simulink model "OutputMVA"  (Simulink 8.7)
settings: Solver=ode45  StartTime=0.0  StopTime=10.0  RelTol=1e-3
undefined symbols (not defined in the file or in its folder): sMP
(part 3 of 3)

== system OutputMVA/OutputMVA_ACM/AMA_Filter ==
  NOx_gas_in : Inport
  Gain : Gain
  NOx_filtered : Outport
  wires:
  Gain/1 -> NOx_filtered/1
  NOx_gas_in/1 -> Gain/1

== system OutputMVA/OutputMVA_ACM/AMA_Filter1 ==
  NOx_gas_in : Inport
  Gain : Gain
  NOx_filtered : Outport
  wires:
  Gain/1 -> NOx_filtered/1
  NOx_gas_in/1 -> Gain/1

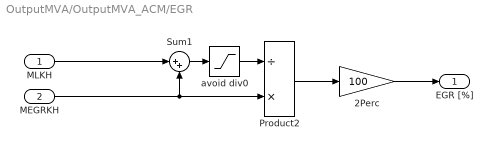
== system OutputMVA/OutputMVA_ACM/EGR ==
  MLKH : Inport
  MEGRKH : Inport  Port=2
  2Perc : Gain  Gain=100
  Product2 : Product  Inputs=/*  RndMeth=Zero
  Sum1 : Sum  Inputs=|++
  avoid div0 : Saturate  UpperLimit=inf  LowerLimit=0.000001
  "EGR [%] " : Outport
  wires:
  avoid div0/1 -> Product2/1
  2Perc/1 -> "EGR [%] "/1
  Sum1/1 -> avoid div0/1
  MLKH/1 -> Sum1/1
  MEGRKH/1 -> Product2/2, Sum1/2
  Product2/1 -> 2Perc/1

== system OutputMVA/OutputMVA_ACM/abs2rel_1 ==
  pressure_absolute : Inport
  Sum : Sum  Inputs=|+-
  pressure_relative : Outport
  wires:
  pressure_absolute/1 -> Sum/1
  Sum/1 -> pressure_relative/1
  [acm_OutputMVA_PressureReference] -> Sum/2

== system OutputMVA/OutputMVA_ACM/abs2rel_11 ==
  pressure_absolute : Inport
  Sum : Sum  Inputs=|+-
  pressure_relative : Outport
  wires:
  [acm_OutputMVA_PressureReference] -> Sum/2
  Sum/1 -> pressure_relative/1
  pressure_absolute/1 -> Sum/1

== system OutputMVA/OutputMVA_ACM/abs2rel_13 ==
  pressure_absolute : Inport
  Sum : Sum  Inputs=|+-
  pressure_relative : Outport
  wires:
  pressure_absolute/1 -> Sum/1
  Sum/1 -> pressure_relative/1
  [acm_OutputMVA_PressureReference] -> Sum/2

== system OutputMVA/OutputMVA_ACM/abs2rel_2 ==
  pressure_absolute : Inport
  Sum : Sum  Inputs=|+-
  pressure_relative : Outport
  wires:
  [acm_OutputMVA_PressureReference] -> Sum/2
  Sum/1 -> pressure_relative/1
  pressure_absolute/1 -> Sum/1

== system OutputMVA/OutputMVA_ACM/abs2rel_3 ==
  pressure_absolute : Inport
  Sum : Sum  Inputs=|+-
  pressure_relative : Outport
  wires:
  [acm_OutputMVA_PressureReference] -> Sum/2
  Sum/1 -> pressure_relative/1
  pressure_absolute/1 -> Sum/1

== system OutputMVA/OutputMVA_ACM/abs2rel_4 ==
  pressure_absolute : Inport
  Sum : Sum  Inputs=|+-
  pressure_relative : Outport
  wires:
  pressure_absolute/1 -> Sum/1
  Sum/1 -> pressure_relative/1
  [acm_OutputMVA_PressureReference] -> Sum/2

== system OutputMVA/OutputMVA_ACM/abs2rel_5 ==
  pressure_absolute : Inport
  Sum : Sum  Inputs=|+-
  pressure_relative : Outport
  wires:
  pressure_absolute/1 -> Sum/1
  Sum/1 -> pressure_relative/1
  [acm_OutputMVA_PressureReference] -> Sum/2

== system OutputMVA/OutputMVA_ACM/abs2rel_6 ==
  pressure_absolute : Inport
  Sum : Sum  Inputs=|+-
  pressure_relative : Outport
  wires:
  [acm_OutputMVA_PressureReference] -> Sum/2
  Sum/1 -> pressure_relative/1
  pressure_absolute/1 -> Sum/1

== system OutputMVA/OutputMVA_ACM/abs2rel_7 ==
  pressure_absolute : Inport
  Sum : Sum  Inputs=|+-
  pressure_relative : Outport
  wires:
  [acm_OutputMVA_PressureReference] -> Sum/2
  Sum/1 -> pressure_relative/1
  pressure_absolute/1 -> Sum/1

== system OutputMVA/OutputMVA_ACM/abs2rel_8 ==
  pressure_absolute : Inport
  Sum : Sum  Inputs=|+-
  pressure_relative : Outport
  wires:
  pressure_absolute/1 -> Sum/1
  Sum/1 -> pressure_relative/1
  [acm_OutputMVA_PressureReference] -> Sum/2

== system OutputMVA/OutputMVA_ACM/abs2rel_9 ==
  pressure_absolute : Inport
  Sum : Sum  Inputs=|+-
  pressure_relative : Outport
  wires:
  pressure_absolute/1 -> Sum/1
  Sum/1 -> pressure_relative/1
  [acm_OutputMVA_PressureReference] -> Sum/2

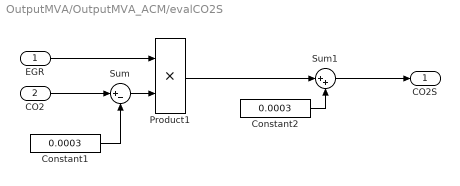
== system OutputMVA/OutputMVA_ACM/evalCO2S ==
  EGR : Inport
  CO2 : Inport  Port=2
  Constant1 : Constant  Value=0.0003
  Constant2 : Constant  Value=0.0003
  Product1 : Product  RndMeth=Zero
  Sum : Sum  Inputs=|+-
  Sum1 : Sum  Inputs=|++
  CO2S : Outport
  wires:
  EGR/1 -> Product1/1
  CO2/1 -> Sum/1
  Sum/1 -> Product1/2
  Constant1/1 -> Sum/2
  Product1/1 -> Sum1/1
  Constant2/1 -> Sum1/2
  Sum1/1 -> CO2S/1

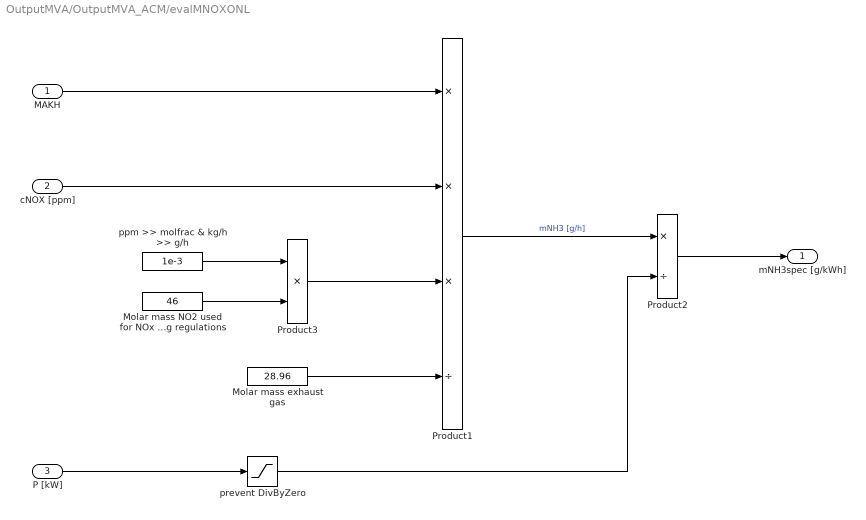
== system OutputMVA/OutputMVA_ACM/evalMNOXONL ==
  MAKH : Inport
  cNOX [ppm] : Inport  Port=2
  P [kW] : Inport  Port=3
  Molar mass NO2 used for NOx according regulations : Constant  Value=46
  Molar mass exhaust gas : Constant  Value=28.96
  Product1 : Product  Inputs=***/  RndMeth=Zero
  Product2 : Product  Inputs=*/  RndMeth=Zero
  Product3 : Product  RndMeth=Zero
  ppm >> molfrac & kg/h >> g/h : Constant  Value=1e-3
  prevent DivByZero : Saturate  UpperLimit=inf  LowerLimit=1e-6
  "mNH3spec [g/kWh] " : Outport
  wires:
  cNOX [ppm]/1 -> Product1/2
  MAKH/1 -> Product1/1
  Product1/1 -> Product2/1  "mNH3 [g/h]"
  Molar mass exhaust gas/1 -> Product1/4
  ppm >> molfrac & kg/h >> g/h/1 -> Product3/1
  Molar mass NO2 used for NOx according regulations/1 -> Product3/2
  Product3/1 -> Product1/3
  Product2/1 -> "mNH3spec [g/kWh] "/1
  P [kW]/1 -> prevent DivByZero/1
  prevent DivByZero/1 -> Product2/2

== system OutputMVA/OutputMVA_ACM/evalPower ==
  n [rpm] : Inport
  M [Nm] : Inport  Port=2
  Product : Product  Inputs=***/  RndMeth=Zero
  const : Constant  Value=30*1000
  pi : Constant  Value=pi
  P [kW] : Outport
  wires:
  pi/1 -> Product/3
  const/1 -> Product/4
  n [rpm]/1 -> Product/1
  M [Nm]/1 -> Product/2
  Product/1 -> P [kW]/1

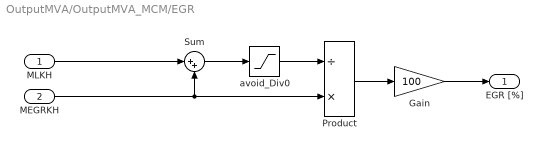
== system OutputMVA/OutputMVA_MCM/EGR ==
  MLKH : Inport
  MEGRKH : Inport  Port=2
  Gain : Gain  Gain=100
  Product : Product  Inputs=/*  RndMeth=Zero
  Sum : Sum  Inputs=|++
  avoid_Div0 : Saturate  UpperLimit=inf  LowerLimit=0.000001
  "EGR [%] " : Outport
  wires:
  Product/1 -> Gain/1
  MEGRKH/1 -> Sum/2, Product/2
  MLKH/1 -> Sum/1
  Sum/1 -> avoid_Div0/1
  avoid_Div0/1 -> Product/1
  Gain/1 -> "EGR [%] "/1

== system OutputMVA/OutputMVA_MCM/abs2rel_1 ==
  pressure_absolute : Inport
  Sum : Sum  Inputs=|+-
  pressure_relative : Outport
  wires:
  [mcm_OutputMVA_PressureReference] -> Sum/2
  Sum/1 -> pressure_relative/1
  pressure_absolute/1 -> Sum/1

== system OutputMVA/OutputMVA_MCM/abs2rel_10 ==
  pressure_absolute : Inport
  Sum : Sum  Inputs=|+-
  pressure_relative : Outport
  wires:
  pressure_absolute/1 -> Sum/1
  Sum/1 -> pressure_relative/1
  [mcm_OutputMVA_PressureReference] -> Sum/2

== system OutputMVA/OutputMVA_MCM/abs2rel_11 ==
  pressure_absolute : Inport
  Sum : Sum  Inputs=|+-
  pressure_relative : Outport
  wires:
  pressure_absolute/1 -> Sum/1
  Sum/1 -> pressure_relative/1
  [mcm_OutputMVA_PressureReference] -> Sum/2

== system OutputMVA/OutputMVA_MCM/abs2rel_12 ==
  pressure_absolute : Inport
  Sum : Sum  Inputs=|+-
  pressure_relative : Outport
  wires:
  pressure_absolute/1 -> Sum/1
  Sum/1 -> pressure_relative/1
  [mcm_OutputMVA_PressureReference] -> Sum/2

== system OutputMVA/OutputMVA_MCM/abs2rel_13 ==
  pressure_absolute : Inport
  Sum : Sum  Inputs=|+-
  pressure_relative : Outport
  wires:
  [mcm_OutputMVA_PressureReference] -> Sum/2
  Sum/1 -> pressure_relative/1
  pressure_absolute/1 -> Sum/1

== system OutputMVA/OutputMVA_MCM/abs2rel_14 ==
  pressure_absolute : Inport
  Sum : Sum  Inputs=|+-
  pressure_relative : Outport
  wires:
  pressure_absolute/1 -> Sum/1
  Sum/1 -> pressure_relative/1
  [mcm_OutputMVA_PressureReference] -> Sum/2

== system OutputMVA/OutputMVA_MCM/abs2rel_15 ==
  pressure_absolute : Inport
  Sum : Sum  Inputs=|+-
  pressure_relative : Outport
  wires:
  pressure_absolute/1 -> Sum/1
  Sum/1 -> pressure_relative/1
  [mcm_OutputMVA_PressureReference] -> Sum/2

== system OutputMVA/OutputMVA_MCM/abs2rel_2 ==
  pressure_absolute : Inport
  Sum : Sum  Inputs=|+-
  pressure_relative : Outport
  wires:
  pressure_absolute/1 -> Sum/1
  Sum/1 -> pressure_relative/1
  [mcm_OutputMVA_PressureReference] -> Sum/2

== system OutputMVA/OutputMVA_MCM/abs2rel_3 ==
  pressure_absolute : Inport
  Sum : Sum  Inputs=|+-
  pressure_relative : Outport
  wires:
  pressure_absolute/1 -> Sum/1
  Sum/1 -> pressure_relative/1
  [mcm_OutputMVA_PressureReference] -> Sum/2

== system OutputMVA/OutputMVA_MCM/abs2rel_4 ==
  pressure_absolute : Inport
  Sum : Sum  Inputs=|+-
  pressure_relative : Outport
  wires:
  [mcm_OutputMVA_PressureReference] -> Sum/2
  Sum/1 -> pressure_relative/1
  pressure_absolute/1 -> Sum/1

== system OutputMVA/OutputMVA_MCM/abs2rel_5 ==
  pressure_absolute : Inport
  Sum : Sum  Inputs=|+-
  pressure_relative : Outport
  wires:
  [mcm_OutputMVA_PressureReference] -> Sum/2
  Sum/1 -> pressure_relative/1
  pressure_absolute/1 -> Sum/1

== system OutputMVA/OutputMVA_MCM/abs2rel_6 ==
  pressure_absolute : Inport
  Sum : Sum  Inputs=|+-
  pressure_relative : Outport
  wires:
  pressure_absolute/1 -> Sum/1
  Sum/1 -> pressure_relative/1
  [mcm_OutputMVA_PressureReference] -> Sum/2

== system OutputMVA/OutputMVA_MCM/abs2rel_7 ==
  pressure_absolute : Inport
  Sum : Sum  Inputs=|+-
  pressure_relative : Outport
  wires:
  pressure_absolute/1 -> Sum/1
  Sum/1 -> pressure_relative/1
  [mcm_OutputMVA_PressureReference] -> Sum/2

== system OutputMVA/OutputMVA_MCM/abs2rel_8 ==
  pressure_absolute : Inport
  Sum : Sum  Inputs=|+-
  pressure_relative : Outport
  wires:
  [mcm_OutputMVA_PressureReference] -> Sum/2
  Sum/1 -> pressure_relative/1
  pressure_absolute/1 -> Sum/1

== system OutputMVA/OutputMVA_MCM/abs2rel_9 ==
  pressure_absolute : Inport
  Sum : Sum  Inputs=|+-
  pressure_relative : Outport
  wires:
  [mcm_OutputMVA_PressureReference] -> Sum/2
  Sum/1 -> pressure_relative/1
  pressure_absolute/1 -> Sum/1

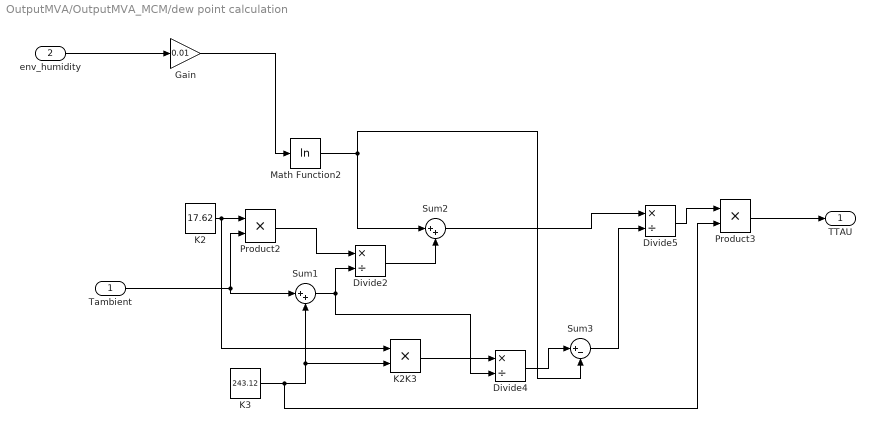
== system OutputMVA/OutputMVA_MCM/dew point calculation ==
  Tambient : Inport
  env_humidity : Inport  Port=2
  Divide2 : Product  Inputs=*/
  Divide4 : Product  Inputs=*/
  Divide5 : Product  Inputs=*/
  Gain : Gain  Gain=0.01
  K2 : Constant  Value=17.62
  K2K3 : Product  RndMeth=Zero
  K3 : Constant  Value=243.12
  Math Function2 : Math  Operator=log  SaturateOnIntegerOverflow=on
  Product2 : Product  RndMeth=Zero
  Product3 : Product  RndMeth=Zero
  Sum1 : Sum  Inputs=|++
  Sum2 : Sum  Inputs=|++
  Sum3 : Sum  Inputs=|+-
  TTAU : Outport
  wires:
  Divide2/1 -> Sum2/2
  Divide4/1 -> Sum3/1
  Divide5/1 -> Product3/1
  K2K3/1 -> Divide4/1
  Tambient/1 -> Product2/2, Sum1/1
  Sum1/1 -> Divide2/2, Divide4/2
  env_humidity/1 -> Gain/1
  Math Function2/1 -> Sum3/2, Sum2/1
  Sum3/1 -> Divide5/2
  Sum2/1 -> Divide5/1
  Product3/1 -> TTAU/1
  Gain/1 -> Math Function2/1
  K2/1 -> K2K3/1, Product2/1
  Product2/1 -> Divide2/1
  K3/1 -> Product3/2, K2K3/2, Sum1/2

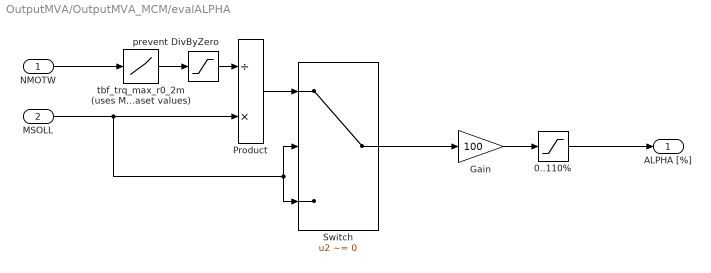
== system OutputMVA/OutputMVA_MCM/evalALPHA ==
  NMOTW : Inport
  MSOLL : Inport  Port=2
  0..110% : Saturate  UpperLimit=110  LowerLimit=0
  Gain : Gain  Gain=100
  Product : Product  Inputs=/*  RndMeth=Zero
  Switch : Switch  Criteria=u2 ~= 0
  prevent DivByZero : Saturate  UpperLimit=inf  LowerLimit=1e-6
  tbf_trq_max_r0_2m (uses MCM dataset values) : Lookup  Description=|  InputValues=sMP.ctrl.mcm.tbf_trq_max_r0_x_eng_speed  Table=sMP.ctrl.mcm.tbf_trq_max_r0_2m  LookUpMeth=Interpolation-Use End Values
      | Look-up table of dSPACE TargetLink.
      | 
      | This block calculates the output values dependant on the given characteristic. Note that the vector of input values must be monotonically increasing for TargetLink.
  ALPHA [%] : Outport
  wires:
  Switch/1 -> Gain/1
  Product/1 -> Switch/1
  0..110%/1 -> ALPHA [%]/1
  Gain/1 -> 0..110%/1
  MSOLL/1 -> Switch/3, Switch/2, Product/2
  NMOTW/1 -> tbf_trq_max_r0_2m (uses MCM dataset values)/1
  tbf_trq_max_r0_2m (uses MCM dataset values)/1 -> prevent DivByZero/1
  prevent DivByZero/1 -> Product/1

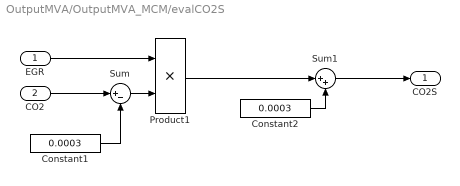
== system OutputMVA/OutputMVA_MCM/evalCO2S ==
  EGR : Inport
  CO2 : Inport  Port=2
  Constant1 : Constant  Value=0.0003
  Constant2 : Constant  Value=0.0003
  Product1 : Product  RndMeth=Zero
  Sum : Sum  Inputs=|+-
  Sum1 : Sum  Inputs=|++
  CO2S : Outport
  wires:
  Sum1/1 -> CO2S/1
  Constant2/1 -> Sum1/2
  Product1/1 -> Sum1/1
  Constant1/1 -> Sum/2
  Sum/1 -> Product1/2
  CO2/1 -> Sum/1
  EGR/1 -> Product1/1

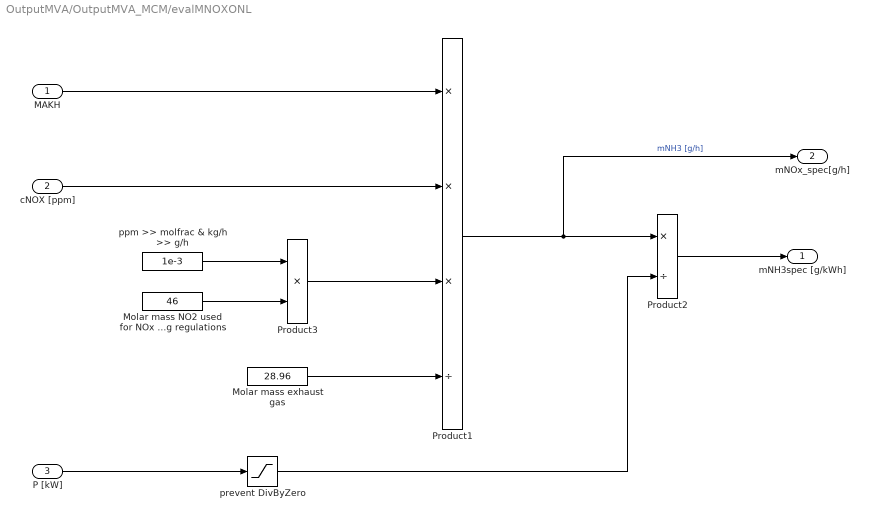
== system OutputMVA/OutputMVA_MCM/evalMNOXONL ==
  MAKH : Inport
  cNOX [ppm] : Inport  Port=2
  P [kW] : Inport  Port=3
  Molar mass NO2 used for NOx according regulations : Constant  Value=46
  Molar mass exhaust gas : Constant  Value=28.96
  Product1 : Product  Inputs=***/  RndMeth=Zero
  Product2 : Product  Inputs=*/  RndMeth=Zero
  Product3 : Product  RndMeth=Zero
  ppm >> molfrac & kg/h >> g/h : Constant  Value=1e-3
  prevent DivByZero : Saturate  UpperLimit=inf  LowerLimit=1e-6
  "mNH3spec [g/kWh] " : Outport
  mNOx_spec[g/h] : Outport  Port=2
  wires:
  prevent DivByZero/1 -> Product2/2
  P [kW]/1 -> prevent DivByZero/1
  Product2/1 -> "mNH3spec [g/kWh] "/1
  Product3/1 -> Product1/3
  Molar mass NO2 used for NOx according regulations/1 -> Product3/2
  ppm >> molfrac & kg/h >> g/h/1 -> Product3/1
  Molar mass exhaust gas/1 -> Product1/4
  Product1/1 -> mNOx_spec[g/h]/1, Product2/1  "mNH3 [g/h]"
  MAKH/1 -> Product1/1
  cNOX [ppm]/1 -> Product1/2

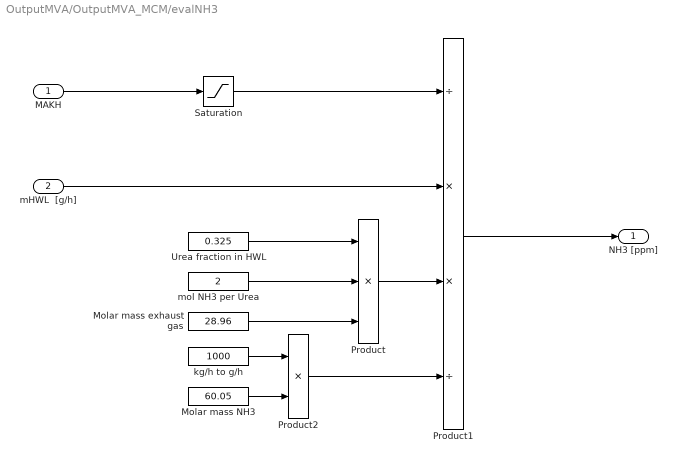
== system OutputMVA/OutputMVA_MCM/evalNH3 ==
  MAKH : Inport
  mHWL  [g/h] : Inport  Port=2
  Molar mass NH3 : Constant  Value=60.05
  Molar mass exhaust gas : Constant  Value=28.96
  Product : Product  Inputs=3  RndMeth=Zero
  Product1 : Product  Inputs=/**/  RndMeth=Zero
  Product2 : Product  RndMeth=Zero
  Saturation : Saturate  UpperLimit=inf  LowerLimit=0
  Urea fraction in HWL : Constant  Value=0.325
  kg/h to g/h : Constant  Value=1000
  mol NH3 per Urea : Constant  Value=2
  "NH3 [ppm] " : Outport
  wires:
  mol NH3 per Urea/1 -> Product/2
  Molar mass exhaust gas/1 -> Product/3
  Molar mass NH3/1 -> Product2/2
  kg/h to g/h/1 -> Product2/1
  Urea fraction in HWL/1 -> Product/1
  Product2/1 -> Product1/4
  Product/1 -> Product1/3
  Product1/1 -> "NH3 [ppm] "/1
  MAKH/1 -> Saturation/1
  mHWL  [g/h]/1 -> Product1/2
  Saturation/1 -> Product1/1

== system OutputMVA/OutputMVA_MCM/evalP3 ==
  P31 : Inport
  P32 : Inport  Port=2
  Add : Sum
  Gain : Gain  Gain=0.5
  P3 : Outport
  wires:
  P32/1 -> Add/2
  Gain/1 -> P3/1
  P31/1 -> Add/1
  Add/1 -> Gain/1

== system OutputMVA/OutputMVA_MCM/evalPower ==
  n [rpm] : Inport
  M [Nm] : Inport  Port=2
  Product : Product  Inputs=***/  RndMeth=Zero
  const : Constant  Value=30*1000
  pi : Constant  Value=pi
  P [kW] : Outport
  wires:
  Product/1 -> P [kW]/1
  M [Nm]/1 -> Product/2
  n [rpm]/1 -> Product/1
  const/1 -> Product/4
  pi/1 -> Product/3

== system OutputMVA/OutputMVA_MCM/evalT3 ==
  In1 : Inport
  In2 : Inport  Port=2
  Add : Sum
  Gain : Gain  Gain=0.5
  Out : Outport
  wires:
  In2/1 -> Add/2
  Gain/1 -> Out/1
  In1/1 -> Add/1
  Add/1 -> Gain/1
